simulink library "dlbsBlockMean"  (R2025b)
settings: Solver=VariableStepAuto  StartTime=0.0  StopTime=10.0  RelTol=1e-3
libraries: dlbsBlockExtractGradientGF x1, dlbsBlockInsertGradientGF x1
settings Model: Creator=lt6037  LastModifiedBy=lt6037

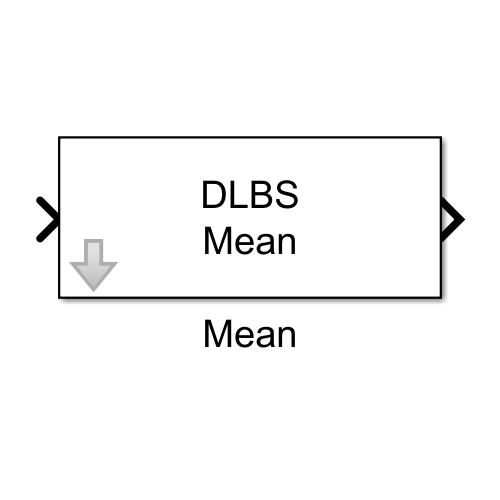
[thumbnail: Simulink's stored preview of the top-level diagram]
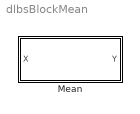
== system dlbsBlockMean ==
  Mean : Subsystem
      mask help: Computes the arithmetic mean over all elements of an input tensor, producing a scalar output.
      mask Help: web("dlbsHelpBlockMean.html")
      mask Display: fprintf("DLBS\nMean")

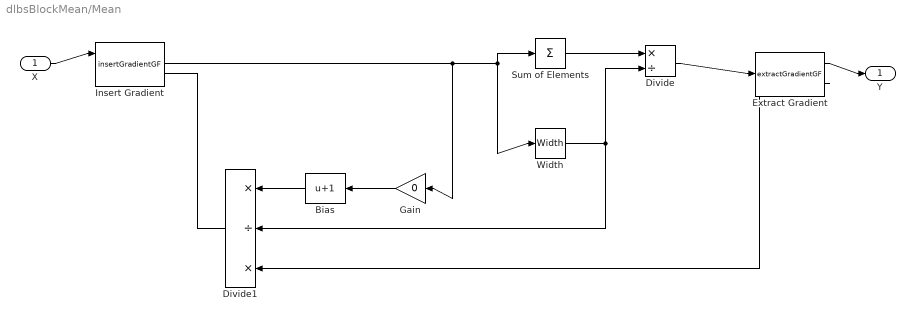
== system dlbsBlockMean/Mean ==
  X : Inport
  Bias : Bias  Bias=1  SaturateOnIntegerOverflow=off
  Divide : Product  Inputs=*/
  Divide1 : Product  Inputs=*/*
  Extract Gradient : dlbsBlockExtractGradientGF/extractGradientGF
  Gain : Gain  Gain=0
  Insert Gradient : dlbsBlockInsertGradientGF/insertGradientGF
  Sum of Elements : Sum  Inputs=+
  Width : Width
  Y : Outport
  wires:
  Insert Gradient/1 -> Gain/1, Width/1, Sum of Elements/1
  Divide/1 -> Extract Gradient/1
  Sum of Elements/1 -> Divide/1
  Width/1 -> Divide/2, Divide1/2
  Gain/1 -> Bias/1
  Bias/1 -> Divide1/1
  Divide1/1 -> Insert Gradient/2
  Extract Gradient/2 -> Divide1/3
  X/1 -> Insert Gradient/1
  Extract Gradient/1 -> Y/1
